simulink model "controllo_SS_no_obs2023b"  (R2023b)
settings: Solver=VariableStepAuto  StartTime=0.0  StopTime=20.0  RelTol=1e-3
values from neighbouring files (symbols this model uses):
  Ken_eta = K(:, 4)    [LQ_KF.m]    (also in LQ_KF_version1.m; LQ_KF_version2.m = Ken(:, n+1:end); LQ_Luenberger.m; LQ_prova.m = Ken(:, n+1:end))
  Ken_x = K(:, 1:3)    [LQ_KF.m]    (also in LQ_KF_version1.m; LQ_KF_version2.m = Ken(:, 1:n); LQ_Luenberger.m; LQ_prova.m = Ken(:, 1:n))
undefined symbols (not defined in the file or in its folder): Lc, Rtot, x1_eq0, x2_eq0, x3_eq0
libraries: simulink x1
settings Model: Creator=Pronto all'uso  LastModifiedBy=Pronto all'uso

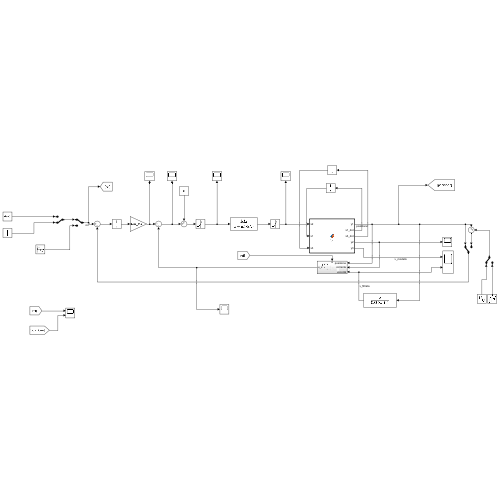
[thumbnail: Simulink's stored preview of the top-level diagram]
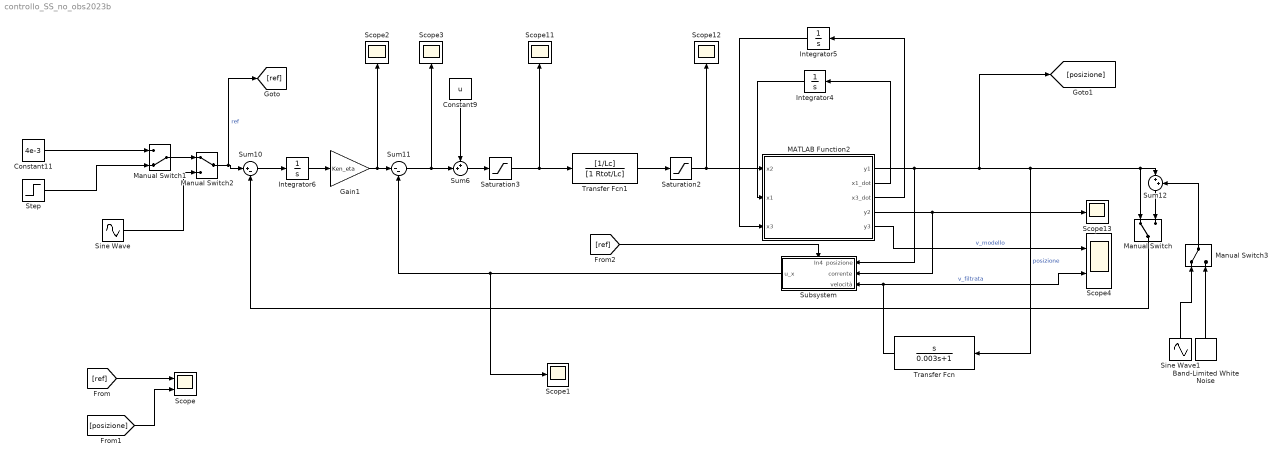
== system controllo_SS_no_obs2023b ==
  Band-Limited White Noise : simulink/Sources/Band-Limited White Noise  Cov=[8.9934e-11*0.002]  Ts=0.002  seed=[23341]
  Constant11 : Constant  Value=4e-3
  Constant9 : Constant  Value=u
  Gain1 : Gain  Gain=Ken_eta
  Integrator4 : Integrator
  Integrator5 : Integrator
  Integrator6 : Integrator
  MATLAB Function2 : MATLAB Function  TreatAsAtomicUnit=on
  Manual Switch : ManualSwitch
  Manual Switch1 : ManualSwitch  CurrentSetting=0
  Manual Switch2 : ManualSwitch
  Manual Switch3 : ManualSwitch
  Saturation2 : Saturate  UpperLimit=3  LowerLimit=0
  Saturation3 : Saturate  UpperLimit=24  LowerLimit=-24
  Scope : Scope  NumInputPorts=2
  Scope{1..3,11..13} (6 alike) : Scope
  Scope4 : Scope  NumInputPorts=2
  Sine Wave : Sin  Amplitude=0.001  Bias=0.004  Frequency=4  SampleTime=0
  Sine Wave1 : Sin  Amplitude=0.00001  Frequency=50  SampleTime=0.002
  Step : Step  After=0.006  SampleTime=0
  Subsystem : Subsystem
      settings: PortSchema="{\"entries\":[{\"content\":{\"sides\":[{\"content\":{\"connectorIds\":[\"In1\",\"In2\",\"In3\"]},\"type\":\"ConnectorPlacement.EquallySpacedRectSide\",\"uuid\":\"c1bcbe62-bd51-4340-8372-7adb28c30fc3\"},{\"content\":{\"connectorIds\":[\"Out1\"],\"side\":\"RIGHT\"},\"type\":\"ConnectorPlacement.EquallySpacedRectSide\",\"uuid\":\"b887fdbd-6521-478b-ab36-0ec54fcd91d0\"},{\"content\":{\"connectorIds\":[\"In4\"],\"side\":\"TOP\"},\"type\":\"ConnectorPlacement.EquallySpacedRectSide\",\"uuid\":\"ecc58360-309a-4020-bddd-fd047277d90d\"}]},\"type\":\"ConnectorPlacement.EquallySpacedConnector\",\"uuid\":\"0c91a21a-ebab-4362-8b63-826f56475d15\"}],\"packageUris\":[\"http://schema.mathworks.com/mf0/Connector/R2020b\"],\"version\":\"1.0\"}"
  Sum10 : Sum  Inputs=|+-
  Sum11 : Sum  Inputs=|--
  Sum12 : Sum  Inputs=|++
  Sum6 : Sum  Inputs=++|
  Transfer Fcn : TransferFcn  Numerator=[1 0]  Denominator=[0.003 1]
  Transfer Fcn1 : TransferFcn  Numerator=[1/Lc]  Denominator=[1 Rtot/Lc]
  wires:
  Integrator5/1 -> MATLAB Function2/3(x3)
  MATLAB Function2/3(x3_dot) -> Integrator5/1
  Transfer Fcn1/1 -> Saturation2/1
  Sum11/1 -> Scope3/1, Sum6/2
  Integrator6/1 -> Gain1/1
  Manual Switch3/1 -> Sum12/2
  Saturation2/1 -> MATLAB Function2/1(x2), Scope12/1
  Manual Switch1/1 -> Manual Switch2/1
  Sum6/1 -> Saturation3/1
  MATLAB Function2/1(y1) -> Subsystem/1(posizione), [posizione], Transfer Fcn/1, Sum12/1, Manual Switch/1  "posizione"
  Sum12/1 -> Manual Switch/2
  Band-Limited White Noise/1 -> Manual Switch3/2
  Integrator4/1 -> MATLAB Function2/2(x1)
  Sine Wave/1 -> Manual Switch2/2
  MATLAB Function2/4(y2) -> Subsystem/2(corrente), Scope13/1
  Manual Switch2/1 -> [ref], Sum10/1  "ref"
  Constant9/1 -> Sum6/1
  Gain1/1 -> Sum11/1, Scope2/1
  Sine Wave1/1 -> Manual Switch3/1
  MATLAB Function2/2(x1_dot) -> Integrator4/1
  Sum10/1 -> Integrator6/1
  Saturation3/1 -> Transfer Fcn1/1, Scope11/1
  MATLAB Function2/5(y3) -> Scope4/1  "v_modello"
  Subsystem/1(u_x) -> Scope1/1, Sum11/2
  Manual Switch/1 -> Sum10/2
  [ref] -> Scope/1
  [posizione] -> Scope/2
  Constant11/1 -> Manual Switch1/1
  Step/1 -> Manual Switch1/2
  [ref] -> Subsystem/4(In4)
  Transfer Fcn/1 -> Subsystem/3(velocità), Scope4/2  "v_filtrata"

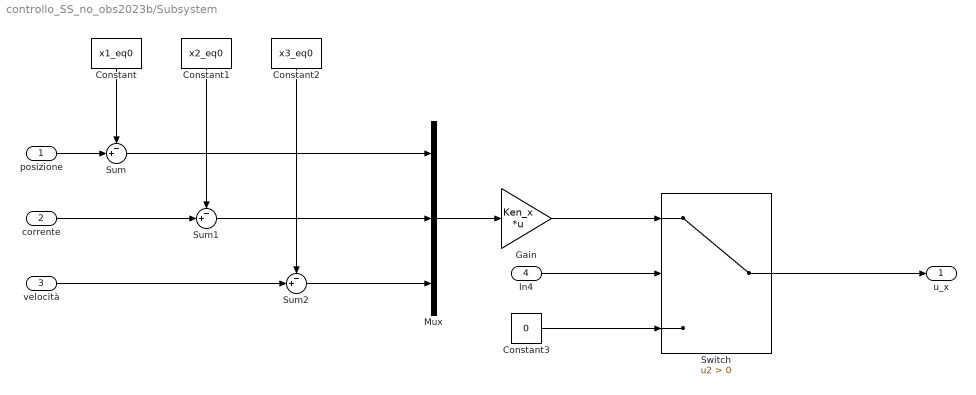
== system controllo_SS_no_obs2023b/Subsystem ==
  posizione : Inport
  corrente : Inport  Port=2
  velocità : Inport  Port=3
  In4 : Inport  Port=4
  Constant : Constant  Value=x1_eq0
  Constant1 : Constant  Value=x2_eq0
  Constant2 : Constant  Value=x3_eq0
  Constant3 : Constant  Value=0
  Gain : Gain  Gain=Ken_x  Multiplication=Matrix(K*u) (u vector)
  Mux : Mux  Inputs=3
  Sum : Sum  Inputs=-+|
  Sum1 : Sum  Inputs=-+|
  Sum2 : Sum  Inputs=-+|
  Switch : Switch  Criteria=u2 > Threshold  SaturateOnIntegerOverflow=off  InputSameDT=off
  u_x : Outport
  wires:
  Constant/1 -> Sum/1
  posizione/1 -> Sum/2
  Constant1/1 -> Sum1/1
  corrente/1 -> Sum1/2
  Constant2/1 -> Sum2/1
  velocità/1 -> Sum2/2
  Sum/1 -> Mux/1
  Sum2/1 -> Mux/3
  Sum1/1 -> Mux/2
  Mux/1 -> Gain/1
  Gain/1 -> Switch/1
  Constant3/1 -> Switch/3
  Switch/1 -> u_x/1
  In4/1 -> Switch/2

== matlab function controllo_SS_no_obs2023b/MATLAB Function2 ==
  data: y1 output; x2 input; x1_dot output; x1 input; x3 input; x3_dot output; y2 output; y3 output
function [y1,x1_dot, x3_dot, y2, y3] = fcn(x2, x1, x3)
    m = 0.0657;
    g = 9.81;
    k_mag = 2.4405e-05;
    Rtot = 9.7585;
    Lc = 0.3708;
    y0 = 0.012;
    
    x1_dot = x3;
    x3_dot = (k_mag/m)*(x2/(y0-x1))^2 - g;

    if x1 <= 0 && x3_dot < 0
        x1 = 0;
        x3 = 0;
        x3_dot = 0;
    end
y1 = x1;
y2 = x2;
y3 = x3;
